simulink model "Lab1AircraftEPS"  (Simulink 9.2)
settings: Solver=ode3  StartTime=0.0  StopTime=5  RelTol=1e-3  EnableMultiTasking=on
PreLoadFcn:
  | warning off
  | Ts=10e-6;
InitFcn:
  | warning off
  | Ts=10e-6;
undefined symbols (not defined in the file): D1, Delta, sigbuilder_block
libraries: powerlib x91, sps_avr x4, powerlib_extras x4, dspstat3 x4
(part 3 of 3)

== system Lab1AircraftEPS/APU1/Feedback measurements &  main contactor/Contactor ==
  com : Inport
  Ideal Switch : powerlib/Power Electronics/Ideal Switch  Ron=0.001  Lon=0  IC=0  Rs=1e3  Cs=inf  Measurements=off
  Ideal Switch1 : powerlib/Power Electronics/Ideal Switch  Ron=0.001  Lon=0  IC=0  Rs=1e3  Cs=inf  Measurements=off
  Ideal Switch2 : powerlib/Power Electronics/Ideal Switch  Ron=0.001  Lon=0  IC=0  Rs=1e3  Cs=inf  Measurements=off
  A : PMIOPort  Side=Left
  a : PMIOPort  Port=2  Side=Right
  B : PMIOPort  Port=3  Side=Left
  b : PMIOPort  Port=4  Side=Right
  C : PMIOPort  Port=5  Side=Left
  c : PMIOPort  Port=6  Side=Right
  wires:
  com/1 -> Ideal Switch1/1, Ideal Switch2/1, Ideal Switch/1
  connections:
  c/RConn1 -- Ideal Switch2/RConn1
  C/RConn1 -- Ideal Switch2/LConn1
  b/RConn1 -- Ideal Switch1/RConn1
  B/RConn1 -- Ideal Switch1/LConn1
  a/RConn1 -- Ideal Switch/RConn1
  A/RConn1 -- Ideal Switch/LConn1

== system Lab1AircraftEPS/APU2/Feedback measurements &  main contactor/Contactor ==
  com : Inport
  Ideal Switch : powerlib/Power Electronics/Ideal Switch  Ron=0.001  Lon=0  IC=0  Rs=1e3  Cs=inf  Measurements=off
  Ideal Switch1 : powerlib/Power Electronics/Ideal Switch  Ron=0.001  Lon=0  IC=0  Rs=1e3  Cs=inf  Measurements=off
  Ideal Switch2 : powerlib/Power Electronics/Ideal Switch  Ron=0.001  Lon=0  IC=0  Rs=1e3  Cs=inf  Measurements=off
  A : PMIOPort  Side=Left
  a : PMIOPort  Port=2  Side=Right
  B : PMIOPort  Port=3  Side=Left
  b : PMIOPort  Port=4  Side=Right
  C : PMIOPort  Port=5  Side=Left
  c : PMIOPort  Port=6  Side=Right
  wires:
  com/1 -> Ideal Switch1/1, Ideal Switch2/1, Ideal Switch/1
  connections:
  c/RConn1 -- Ideal Switch2/RConn1
  C/RConn1 -- Ideal Switch2/LConn1
  b/RConn1 -- Ideal Switch1/RConn1
  B/RConn1 -- Ideal Switch1/LConn1
  a/RConn1 -- Ideal Switch/RConn1
  A/RConn1 -- Ideal Switch/LConn1

== system Lab1AircraftEPS/Left Engine HV/Feedback measurements &  main contactor/Contactor ==
  com : Inport
  Ideal Switch : powerlib/Power Electronics/Ideal Switch  Ron=0.001  Lon=0  IC=0  Rs=1e3  Cs=inf  Measurements=off
  Ideal Switch1 : powerlib/Power Electronics/Ideal Switch  Ron=0.001  Lon=0  IC=0  Rs=1e3  Cs=inf  Measurements=off
  Ideal Switch2 : powerlib/Power Electronics/Ideal Switch  Ron=0.001  Lon=0  IC=0  Rs=1e3  Cs=inf  Measurements=off
  A : PMIOPort  Side=Left
  a : PMIOPort  Port=2  Side=Right
  B : PMIOPort  Port=3  Side=Left
  b : PMIOPort  Port=4  Side=Right
  C : PMIOPort  Port=5  Side=Left
  c : PMIOPort  Port=6  Side=Right
  wires:
  com/1 -> Ideal Switch1/1, Ideal Switch2/1, Ideal Switch/1
  connections:
  c/RConn1 -- Ideal Switch2/RConn1
  C/RConn1 -- Ideal Switch2/LConn1
  b/RConn1 -- Ideal Switch1/RConn1
  B/RConn1 -- Ideal Switch1/LConn1
  a/RConn1 -- Ideal Switch/RConn1
  A/RConn1 -- Ideal Switch/LConn1

== system Lab1AircraftEPS/Right Engine HV/Feedback measurements &  main contactor/Contactor ==
  com : Inport
  Ideal Switch : powerlib/Power Electronics/Ideal Switch  Ron=0.001  Lon=0  IC=0  Rs=1e3  Cs=inf  Measurements=off
  Ideal Switch1 : powerlib/Power Electronics/Ideal Switch  Ron=0.001  Lon=0  IC=0  Rs=1e3  Cs=inf  Measurements=off
  Ideal Switch2 : powerlib/Power Electronics/Ideal Switch  Ron=0.001  Lon=0  IC=0  Rs=1e3  Cs=inf  Measurements=off
  A : PMIOPort  Side=Left
  a : PMIOPort  Port=2  Side=Right
  B : PMIOPort  Port=3  Side=Left
  b : PMIOPort  Port=4  Side=Right
  C : PMIOPort  Port=5  Side=Left
  c : PMIOPort  Port=6  Side=Right
  wires:
  com/1 -> Ideal Switch1/1, Ideal Switch2/1, Ideal Switch/1
  connections:
  c/RConn1 -- Ideal Switch2/RConn1
  C/RConn1 -- Ideal Switch2/LConn1
  b/RConn1 -- Ideal Switch1/RConn1
  B/RConn1 -- Ideal Switch1/LConn1
  a/RConn1 -- Ideal Switch/RConn1
  A/RConn1 -- Ideal Switch/LConn1

== stateflow chart BPCU/Chart ==
  state C1 [parallel]
    settings: executionOrder=1
    state On
      entry: B1 = 1
    state Off
      entry: B1 = 0;
    (default) -> C1.Off
    C1.Off -> C1.On : [GL && in(S.On)]
    C1.On -> C1.Off : [!GL && in(S.Off)]
  state C3 [parallel]
    settings: executionOrder=2
    state Off
      entry: B3 = 0;
    state On
      entry: B3 = 1
    (default) -> C3.Off
    C3.On -> C3.Off : [!AL && in(S.Off)]
    C3.Off -> C3.On : [((!GR && !AR ) || !GL )  && !in(C4.On) && in(S.On) && AL]
  state C4 [parallel]
    settings: executionOrder=3
    state Off
      entry: B4 = 0;
    state On
      entry: B4 = 1
    (default) -> C4.Off
    C4.Off -> C4.On : [((!GL && !AL) || !GR) && !in(C3.On) && in(S.On) && AR]
    C4.On -> C4.Off : [!AR && in(S.Off)]
  state C2 [parallel]
    settings: executionOrder=4
    state On
      entry: B2 = 1
    state Off
      entry: B2 = 0;
    (default) -> C2.Off
    C2.Off -> C2.On : [GR && in(S.On)]
    C2.On -> C2.Off : [!GR && in(S.Off)]
  state C5 [parallel]
    settings: executionOrder=5
    state Off
      entry: B5 = 0;
    state On
      entry: B5 = 1
    (default) -> C5.Off
    C5.Off -> C5.On : [((!GR && !AL && !AR) || !GL) && in(S.On)]
  state C6 [parallel]
    settings: executionOrder=6
    state On
      entry: B6= 1
    state Off
      entry: B6 = 0;
    (default) -> C6.Off
    C6.Off -> C6.On : [((!GL && !AL && !AR) || !GR) && in(S.On)]
  state S [parallel]
    settings: executionOrder=7
    state On
    state Off
    state Listen
    S.On -> Listen
    Listen -> S.Off : [hasChanged(GL) || hasChanged(GR) || hasChanged(AL) || hasChanged(AR)]
    (default) -> S.Off
    S.Off -> S.On
  data: B1 output double; GL input boolean; B2 output double; B3 output double; B4 output double; B5 output double; B6 output double; GR input boolean; AL input boolean; AR input boolean
  events: tick input RISING_EDGE_EVENT
